simulink model "ASK"  (Simulink 8.9)
settings: Solver=ode45  StartTime=0.0  StopTime=100  RelTol=1e-3  EnableMultiTasking=on
libraries: dsparch4 x1, commrandsrc2 x1
settings Model: Creator=Abhilash  LastModifiedBy=JBlanco
settings OptimizationCC: ExpressionDepthLimit=2147483647
settings DebuggingCC: SolverPrmCheckMsg=warning
settings GRTTargetCC: GeneratePreprocessorConditionals=Use local settings

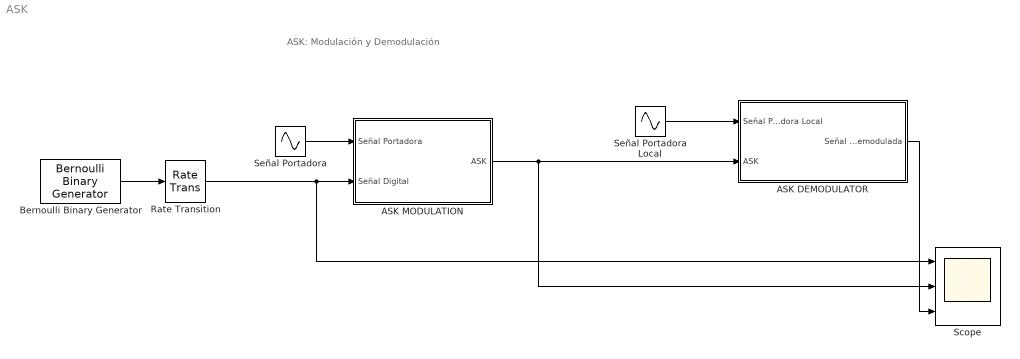
== system ASK ==
  note: ASK: Modulación y Demodulación
  ASK DEMODULATOR : Subsystem
  ASK MODULATION : Subsystem
  Bernoulli Binary Generator : commrandsrc2/Bernoulli Binary Generator  P=0.4  seed=81  Ts=5  frameBased=off  sampPerFrame=1  orient=on  outDataType=double
  Rate Transition : RateTransition  OutPortSampleTime=1/2000
  Scope : Scope  NumInputPorts=3
  Señal Portadora : Sin  Frequency=10*2*pi  Samples=50  SampleTime=1/2000
  Señal Portadora Local : Sin  Frequency=10*2*pi  Samples=50  SampleTime=1/2000
  wires:
  ASK MODULATION/1(ASK) -> Scope/2, ASK DEMODULATOR/2(ASK)
  ASK DEMODULATOR/1(Señal Demodulada) -> Scope/3
  Bernoulli Binary Generator/1 -> Rate Transition/1
  Rate Transition/1 -> Scope/1, ASK MODULATION/2(Señal Digital)
  Señal Portadora/1 -> ASK MODULATION/1(Señal Portadora)
  Señal Portadora Local/1 -> ASK DEMODULATOR/1(Señal Portadora Local)

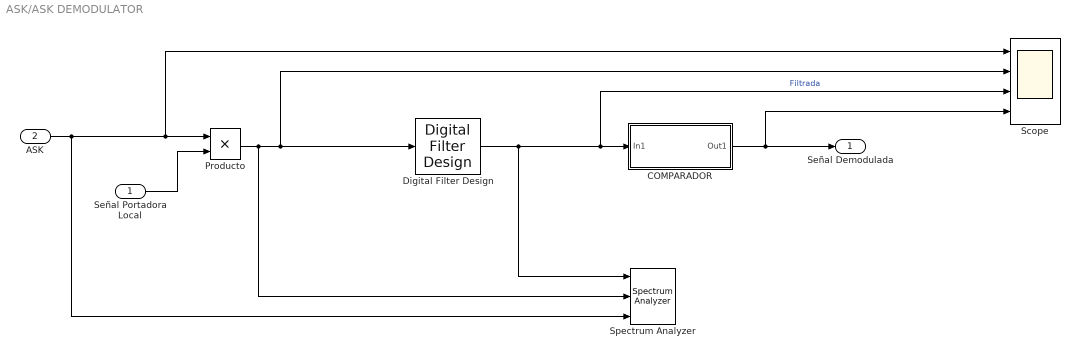
== system ASK/ASK DEMODULATOR ==
  Señal Portadora Local : Inport
  ASK : Inport  Port=2
  COMPARADOR : Subsystem
  Digital Filter Design : dsparch4/Digital Filter Design  mwdsp_browser_bugfix_var=off
  Producto : Product  RndMeth=Zero
  Scope : Scope  NumInputPorts=4
  Spectrum Analyzer : SpectrumAnalyzer  NumInputPorts=3
  Señal Demodulada : Outport
  wires:
  ASK/1 -> Spectrum Analyzer/3, Producto/1, Scope/1
  Señal Portadora Local/1 -> Producto/2
  COMPARADOR/1(Out1) -> Señal Demodulada/1, Scope/4
  Digital Filter Design/1 -> Spectrum Analyzer/1, Scope/3, COMPARADOR/1(In1)  "Filtrada"
  Producto/1 -> Scope/2, Digital Filter Design/1, Spectrum Analyzer/2

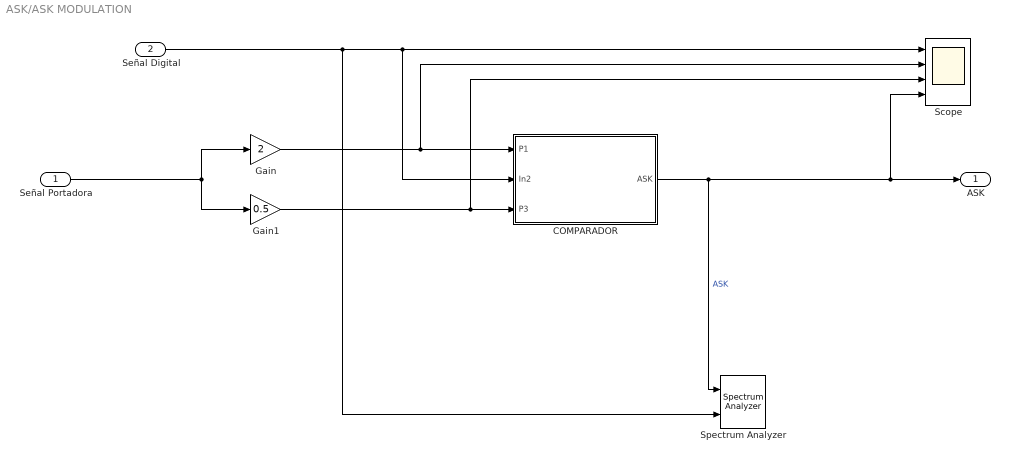
== system ASK/ASK MODULATION ==
  Señal Portadora : Inport
  Señal Digital : Inport  Port=2
  COMPARADOR : Subsystem
  Gain : Gain  Gain=2
  Gain1 : Gain  Gain=0.5
  Scope : Scope  NumInputPorts=4
  Spectrum Analyzer : SpectrumAnalyzer  NumInputPorts=2
  ASK : Outport
  wires:
  Gain/1 -> COMPARADOR/1(P1), Scope/2
  Gain1/1 -> Scope/3, COMPARADOR/3(P3)
  COMPARADOR/1(ASK) -> ASK/1, Scope/4, Spectrum Analyzer/1  "ASK"
  Señal Digital/1 -> Spectrum Analyzer/2, Scope/1, COMPARADOR/2(In2)
  Señal Portadora/1 -> Gain1/1, Gain/1

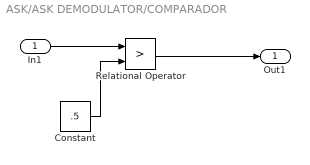
== system ASK/ASK DEMODULATOR/COMPARADOR ==
  In1 : Inport
  Constant : Constant  Value=.5
  Relational Operator : RelationalOperator  Operator=>  OutDataTypeStr=boolean  RndMeth=Nearest
  Out1 : Outport
  wires:
  In1/1 -> Relational Operator/1
  Constant/1 -> Relational Operator/2
  Relational Operator/1 -> Out1/1

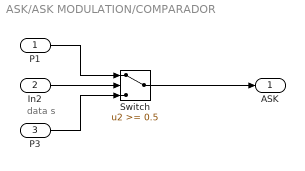
== system ASK/ASK MODULATION/COMPARADOR ==
  note: data s
  P1 : Inport
  In2 : Inport  Port=2
  P3 : Inport  Port=3
  Switch : Switch  Threshold=0.5
  ASK : Outport
  wires:
  P1/1 -> Switch/1
  In2/1 -> Switch/2
  P3/1 -> Switch/3
  Switch/1 -> ASK/1
